simulink model "aero_dap3dof"  (R2021b)
settings: Solver=ode45  StartTime=0  StopTime=300  FixedStep=clockt/4  RelTol=1e-3  AbsTol=1e-6
PreLoadFcn:
  | run('aero_dap3dofdata.m');
undefined symbols (not defined in the file): alph1, alphs1, DB, deg, delt, euler_0, Force, L_arm, mass_0, pqr_0, r_moon_eq, rad, s
libraries: aerolibconvert2 x6, vrlib x2, aerolib6dof2 x1, sharedtransform x1, aerolibutil x1, aerolibgravity2 x1, aero_libdap x1, aero_librcs x1, commchan3 x1
CloseFcn:
  | h=findobj('type','figure','Name','aero_dap3dof');if ~isempty(h);close(h);end
Description:
  | Apollo Lunar Module Digital Autopilot
  | 
  | This model was featured in "Fly Me to the Moon - Then and Now", the story of the digital
  | autopilot in the Lunar Module from the Summer 1999 issue of "MATLAB(R) News & Notes".
  | Double click on the link in the model to view the article online over the Internet.
settings Model: RequirementInfo=9  Creator=The MathWorks, Inc.  LastModifiedBy=dev
settings SolverCC: AutoScaleAbsTol=off  AlgebraicLoopSolver=TrustRegion
settings DataIOCC: SaveFormat=Array  ReturnWorkspaceOutputs=off  SignalLoggingName=logsOut
settings OptimizationCC: BlockReduction=off  ExpressionDepthLimit=2147483647  InitFltsAndDblsToZero=on
settings DebuggingCC: SaveWithParameterizedLinksMsg=none  SignalResolutionControl=TryResolveAllWithWarning  MultiTaskDSMMsg=warning  MultiTaskCondExecSysMsg=none  SigSpecEnsureSampleTimeMsg=none  FcnCallInpInsideContextMsg=warning  StateNameClashWarn=warning  SFUnexpectedBacktrackingDiag=warning  SFNoUnconditionalDefaultTransitionDiag=warning  SFExecutionAtInitializationDiag=none  SFMachineParentedDataDiag=warning  ArithmeticOperatorsInVariantConditions=warning
settings HardwareCC: ProdBitPerPointer=32  ProdBitPerSizeT=32  ProdBitPerPtrDiffT=32  ProdLargestAtomicFloat=None  ProdIntDivRoundTo=Undefined  ProdEndianess=Unspecified  ProdWordSize=32  ProdHWDeviceType=Specified
settings ModelReferenceCC: PropagateSignalLabelsOutOfModel=off
settings SFSimCC: SimUseLocalCustomCode=off  SimParseCustomCode=off  CustomCodeUndefinedFunction=UseInterfaceOnly
settings RTWCC: RTWUseLocalCustomCode=off
settings CodeAppCC: StateflowObjectComments=on
settings GRTTargetCC: TargetLangStandard=C89/C90 (ANSI)
settings ConfigComp: CovMetricSettings=d  CovSaveCumulativeToWorkspaceVar=on  CovSaveSingleToWorkspaceVar=on  CovExternalEMLEnable=off

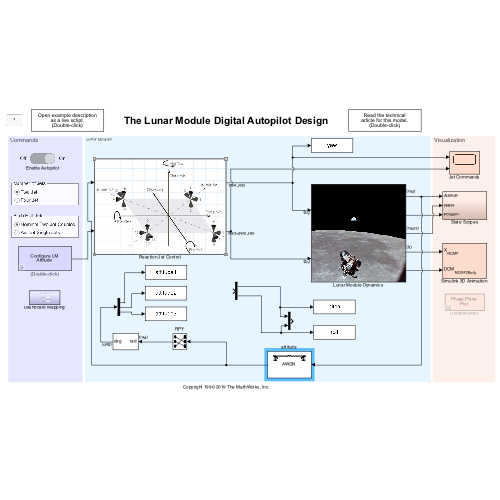
[thumbnail: Simulink's stored preview of the top-level diagram]
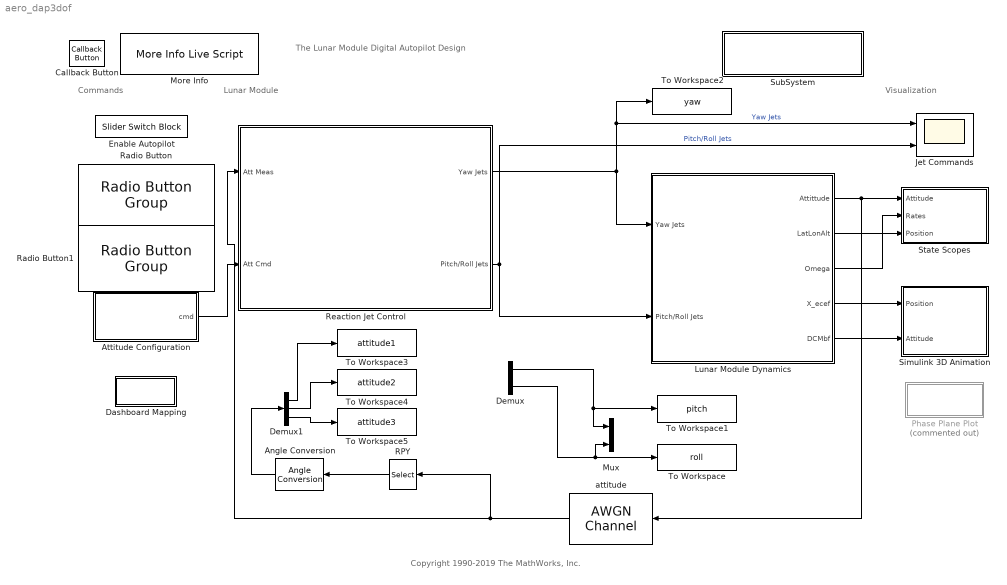
== system aero_dap3dof ==
  note: Lunar Module
  note: Visualization
  note: Commands
  note: The Lunar Module Digital Autopilot Design
  note: Copyright 1990-2019 The MathWorks, Inc.
  Angle Conversion : aerolibconvert2/Angle Conversion  IU=rad  OU=deg
  Attitude Configuration : Subsystem  mask(Configure LM Attitude){att_cmd=euler_0 + [2.87 5.73 0.606], p_0=0.573, q_0=0.573, r_0=6.808}
      mask prompts: att_cmd "<html>Pilot commanded<br>attitude (roll, pitch, yaw)<br>[deg, deg, deg]</html>"; p_0 "Roll rate [deg/s]"; q_0 "Pitch rate [deg/s]"; r_0 "Yaw rate [deg/s]"
      settings: AttributesFormatString=(Double-click)
      mask Callback p_0:
      | assignin('base', 'pqr_0', [str2double(get_param(gcb, 'p_0')),...
      |     str2double(get_param(gcb, 'q_0')), str2double(get_param(gcb, 'r_0'))]);
      mask Callback q_0:
      | assignin('base', 'pqr_0', [str2double(get_param(gcb, 'p_0')),...
      |     str2double(get_param(gcb, 'q_0')), str2double(get_param(gcb, 'r_0'))]);
      mask Callback r_0:
      | assignin('base', 'pqr_0', [str2double(get_param(gcb, 'p_0')),...
      |     str2double(get_param(gcb, 'q_0')), str2double(get_param(gcb, 'r_0'))]);
      mask DialogControl DescGroupVar1 Prompt: Pilot Commanded Body Attitude
      mask DialogControl DescTextVar_copy Prompt: Specify desired body attitude angles to send to digital autopilot.
      mask DialogControl ParameterGroupVar Prompt: Initial Body Angular Rates
      mask DialogControl DescTextVar Prompt: Vary the initial angular rates of the Lunar Module to investigate the response of the digital autopilot design.
      mask Display: disp('Configure LM\nAttitude')
  Callback Button : CallbackButton  ButtonText=?
      settings: ClickFcn=showExample('simulink_aerospace/DevelopingTheApolloLunarModuleDigitalAutopilotExample')
  Dashboard Mapping : Subsystem
  Demux : Demux  Outputs=2
  Demux1 : Demux  Outputs=3
  Enable Autopilot : SliderSwitchBlock  LabelPosition=Hide
      settings: Values={{'Off', 'On'}, [0 1]}
  Jet Commands : Scope  NumInputPorts=2
  Lunar Module Dynamics : Subsystem
      mask Display: image('$imagefile'); % Use "Edit Image" on toolstrip to change.
  More Info : aero_libdap/More Info Live Script  SystemSampleTime=-1  VariantActivationTime=update diagram  Latency=0  AutoFrameSizeCalculation=off
      settings: SourceProductBaseCode=SL
  Mux : Mux  Inputs=2
  Phase Plane Plot : Subsystem  Commented=on  mask(Phase Plane Plot){enablePlot=off}
      mask prompts: enablePlot "Enable yaw phase plane plot"
      mask help: Enable yaw phase plane plotting during simulation.
      settings: AttributesFormatString=(Double-click)
      settings: OpenFcn=|
      | if ~builtin('license','test','virtual_reality_toolbox')
      |     set_param(gcb, 'enableVis', 'off');
      | end
      | open_system(gcb,'mask');
      mask Callback enablePlot:
      | if strcmp(get_param(gcb,'enablePlot'), 'on')
      |     set_param(gcb, 'Commented', 'off');
      | else
      |     set_param(gcb, 'Commented', 'on');
      | end
      mask Display: disp('Phase Plane\nPlot')
  RPY : Selector  InputPortWidth=3  IndexOptions=Index vector (dialog)  Indices=[2 3 1]  OutputSizes=1
  Radio Button : RadioButtonGroup  LabelPosition=Hide  SelectedLabel=Two Jet  ButtonGroupName=Number of Jets
      settings: Values={{'Two Jet', 'Four Jet'}, [2 4]}
  Radio Button1 : RadioButtonGroup  LabelPosition=Hide  SelectedLabel=Nominal Two Jet Couples  ButtonGroupName=Pitch Roll Jets
      settings: Values={{'Nominal Two Jet Couples', 'Ascent Single Jets'}, [2 1]}
  Reaction Jet Control : Subsystem
      mask Display: image('$imagefile'); % Use "Edit Image" on toolstrip to change.
  Simulink 3D Animation : Subsystem  mask(Set Animation Properties){enableVis=on, visSampleTime=1}
      mask prompts: enableVis "Enable visualization with Simulink 3D Animation"; visSampleTime "Animation refresh rate:"
      mask help:
      | Change visualization properties used by Simulink 3D Animation. These settings are graphical only and do not affect simulation behavior.
      |
      | Hover over a dialog box for an explanation of the property.
      settings: OpenFcn=|
      | if ~builtin('license','test','virtual_reality_toolbox')
      |     set_param(gcb, 'enableVis', 'off');
      | end
      | open_system(gcb,'mask');
      mask Callback enableVis:
      | if strcmp(get_param(gcb,'enableVis'), 'on')
      |     enable = {'on', 'on'};
      |     set_param(gcb, 'Commented', 'off');
      | else
      |     enable = {'on', 'off'};
      |     set_param(gcb, 'Commented', 'on');
      | end
      | set_param(gcb,'MaskEnables', enable);
      | clear enable
      mask DialogControl vrOpenBtn Prompt: Open Simulink 3D Animation window
      mask DialogControl vrOpenBtn Callback: vrmfunc('FnOpen',getSimulinkBlockHandle([gcb '/VR Sink']));
      mask DialogControl visSampleTime Tooltip: <html>Sample time of animation window. Use this property to effectively speed up or slow down the animation. For example, a sample time of 1 causes the animation to update at every simulation time step. For a sample time of 20, the visualization will update every twentieth simulation time step. Maximum value is 1000.</html>
      mask Display:
      | port_label('input', 1, 'X_{MCMF}','texmode','on')
      | port_label('input', 2, 'DCM_{MCMF2Body}','texmode','on')
  State Scopes : Subsystem
  SubSystem : Subsystem
      mask init:
      | dispstr = sprintf('Read the technical\narticle for this model.\n(Double-click)');
      settings: OpenFcn=web('https://www.mathworks.com/company/newsletters/articles/the-apollo-11-moon-landing-spacecraft-design-then-and-now.html')
      mask Display: disp(dispstr)
  To Workspace : ToWorkspace  VariableName=roll  SampleTime=-1
      settings: Save2DSignal=2-D array (concatenate along first dimension)
  To Workspace1 : ToWorkspace  VariableName=pitch  SampleTime=-1
      settings: Save2DSignal=2-D array (concatenate along first dimension)
  To Workspace2 : ToWorkspace  VariableName=yaw  SampleTime=-1
      settings: Save2DSignal=2-D array (concatenate along first dimension)
  To Workspace3 : ToWorkspace  VariableName=attitude1  SampleTime=-1
      settings: Save2DSignal=2-D array (concatenate along first dimension)
  To Workspace4 : ToWorkspace  VariableName=attitude2  SampleTime=-1
  To Workspace5 : ToWorkspace  VariableName=attitude3  SampleTime=-1
      settings: Save2DSignal=2-D array (concatenate along first dimension)
  attitude : commchan3/AWGN Channel  InputProcessing=Columns as channels (frame based)  seed=67  noiseMode=Variance from mask  EbNodB=10  EsNodB=10  SNRdB=10  bitsPerSym=1  Ps=1  Tsym=1  variance=0.0000001
  wires:
  Attitude Configuration/1(cmd) -> Reaction Jet Control/2(Att Cmd)
  Lunar Module Dynamics/3(Omega) -> State Scopes/2(Rates)
  Lunar Module Dynamics/4(X_ecef) -> Simulink 3D Animation/1(Position)
  Lunar Module Dynamics/5(DCMbf) -> Simulink 3D Animation/2(Attitude)
  Reaction Jet Control/2(Pitch/Roll Jets) -> Lunar Module Dynamics/2(Pitch/Roll Jets), Jet Commands/2  "Pitch/Roll Jets"
  Demux/1 -> Mux/1, To Workspace1/1
  Lunar Module Dynamics/2(LatLonAlt) -> State Scopes/3(Position)
  Demux/2 -> Mux/2, To Workspace/1
  Lunar Module Dynamics/1(Attittude) -> State Scopes/1(Attitude), attitude/1
  RPY/1 -> Angle Conversion/1
  Angle Conversion/1 -> Demux1/1
  Reaction Jet Control/1(Yaw Jets) -> Lunar Module Dynamics/1(Yaw Jets), Jet Commands/1, To Workspace2/1  "Yaw Jets"
  attitude/1 -> Reaction Jet Control/1(Att Meas), RPY/1
  Demux1/1 -> To Workspace3/1
  Demux1/2 -> To Workspace4/1
  Demux1/3 -> To Workspace5/1

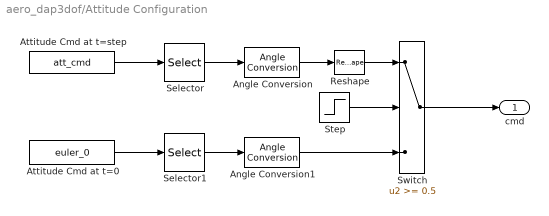
== system aero_dap3dof/Attitude Configuration ==
  Angle Conversion : aerolibconvert2/Angle Conversion  IU=deg  OU=rad
  Angle Conversion1 : aerolibconvert2/Angle Conversion  IU=deg  OU=rad
  Attitude Cmd at t=0 : Constant  Value=euler_0  VectorParams1D=off
  Attitude Cmd at t=step : Constant  Value=att_cmd  VectorParams1D=off
  Reshape : Reshape
  Selector : Selector  InputPortWidth=3  IndexOptions=Index vector (dialog)  Indices=[3 1 2]  OutputSizes=1
  Selector1 : Selector  InputPortWidth=3  IndexOptions=Index vector (dialog)  Indices=[3 1 2]  OutputSizes=1
  Step : Step  Time=.25  SampleTime=0
  Switch : Switch  Threshold=0.5  SaturateOnIntegerOverflow=on  InputSameDT=on
  cmd : Outport  VectorParamsAs1DForOutWhenUnconnected=off
  wires:
  Reshape/1 -> Switch/1
  Angle Conversion/1 -> Reshape/1
  Step/1 -> Switch/2
  Attitude Cmd at t=0/1 -> Selector1/1
  Selector/1 -> Angle Conversion/1
  Switch/1 -> cmd/1
  Selector1/1 -> Angle Conversion1/1
  Angle Conversion1/1 -> Switch/3
  Attitude Cmd at t=step/1 -> Selector/1

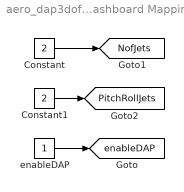
== system aero_dap3dof/Dashboard Mapping ==
  Constant : Constant  Value=2
  Constant1 : Constant  Value=2
  enableDAP : Constant
  tag scope: NofJets=global, PitchRollJets=global, enableDAP=global
  wires:
  Constant/1 -> [NofJets]
  Constant1/1 -> [PitchRollJets]
  enableDAP/1 -> [enableDAP]

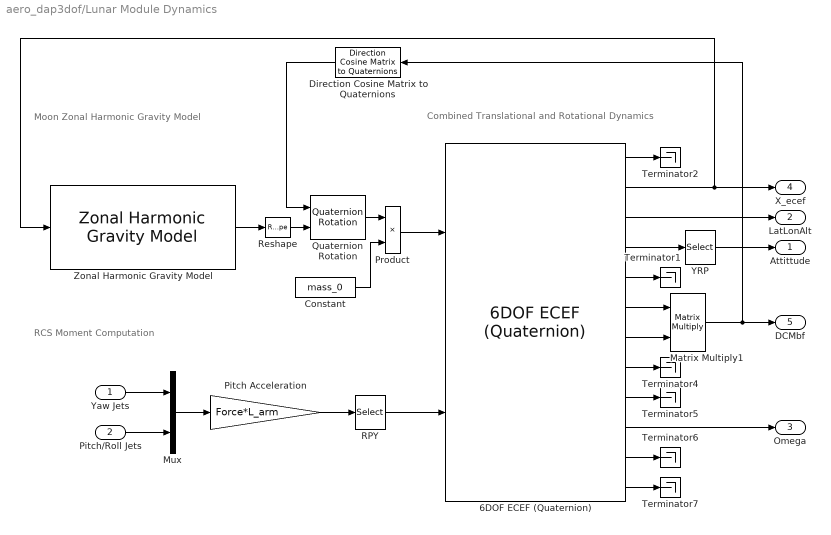
== system aero_dap3dof/Lunar Module Dynamics ==
  note: RCS Moment Computation
  note: Combined Translational and Rotational Dynamics
  note: Moon Zonal Harmonic Gravity Model
  Yaw Jets : Inport  Unit=lbf
  Pitch/Roll Jets : Inport  Port=2  Unit=lbf
  6DOF ECEF (Quaternion) : aerolib6dof2/6DOF ECEF (Quaternion)  units=English (Velocity in ft/s)  mtype=Fixed  xg_0=lla_0  Vm_0=vel_0  eul_0=euler_0*pi/180  pm_0=pqr_0*pi/180  mass_0=mass_0  mass_e=0.5  mass_f=2.0  inertia=Inertia_0  inertia_e=eye(3)  inertia_f=2*eye(3)  vre_flag=on  abi_flag=off  ptype=Custom  R=r_moon_eq  F=f_moon  w_E=omega_moon  angle_in=Internal  LG0=0  quat_statename=''  pm_statename=''  Vm_statename=''  posECEF_statename=''  posECI_statename=''  LG_statename=''  mass_statename=''
      settings: SourceProductBaseCode=AE
  Constant : Constant  Value=mass_0
  Direction Cosine Matrix to Quaternions : sharedtransform/Direction Cosine Matrix  to Quaternions  aMode=0  action=None  tolerance=eps(2)
      settings: SourceProductBaseCode=AE,PW,DR,MT,UV,VE
  Matrix Multiply1 : Product  Multiplication=Matrix(*)
  Mux : Mux  Inputs=2
  Pitch Acceleration : Gain  Gain=Force*L_arm  SaturateOnIntegerOverflow=on  OutDataTypeStr=Inherit: Same as input  ParamDataTypeStr=Inherit: Same as input
  Product : Product
  Quaternion Rotation : aerolibutil/Quaternion Rotation
  RPY : Selector  InputPortWidth=3  IndexOptions=Index vector (dialog)  Indices=[2 3 1]  OutputSizes=1
  Reshape : Reshape
  Terminator{1..2,4..7} (6 alike) : Terminator
  YRP : Selector  InputPortWidth=3  IndexOptions=Index vector (dialog)  Indices=[3 1 2]  OutputSizes=1
  Zonal Harmonic Gravity Model : aerolibgravity2/Zonal Harmonic Gravity Model  units=English  degree=2  action=Warning  ptype=Moon  R=5702099.7375  GM=173140712687447.5  jvalue=[2.0270000e-04]
      settings: SourceProductBaseCode=AE
  Attittude : Outport  Unit=rad  VectorParamsAs1DForOutWhenUnconnected=off
  LatLonAlt : Outport  Port=2  VectorParamsAs1DForOutWhenUnconnected=off
  Omega : Outport  Port=3  Unit=rad/s  VectorParamsAs1DForOutWhenUnconnected=off
  X_ecef : Outport  Port=4  Unit=ft  VectorParamsAs1DForOutWhenUnconnected=off
  DCMbf : Outport  Port=5  VectorParamsAs1DForOutWhenUnconnected=off
  wires:
  Pitch/Roll Jets/1 -> Mux/2
  Yaw Jets/1 -> Mux/1
  Mux/1 -> Pitch Acceleration/1
  6DOF ECEF (Quaternion)/4 -> YRP/1
  6DOF ECEF (Quaternion)/10 -> Omega/1
  Matrix Multiply1/1 -> Direction Cosine Matrix to Quaternions/1, DCMbf/1
  6DOF ECEF (Quaternion)/6 -> Matrix Multiply1/1
  6DOF ECEF (Quaternion)/7 -> Matrix Multiply1/2
  Zonal Harmonic Gravity Model/1 -> Reshape/1
  Quaternion Rotation/1 -> Product/1
  Reshape/1 -> Quaternion Rotation/2
  Direction Cosine Matrix to Quaternions/1 -> Quaternion Rotation/1
  6DOF ECEF (Quaternion)/1 -> Terminator2/1
  6DOF ECEF (Quaternion)/5 -> Terminator1/1
  6DOF ECEF (Quaternion)/2 -> X_ecef/1, Zonal Harmonic Gravity Model/1
  6DOF ECEF (Quaternion)/9 -> Terminator5/1
  6DOF ECEF (Quaternion)/8 -> Terminator4/1
  6DOF ECEF (Quaternion)/11 -> Terminator6/1
  6DOF ECEF (Quaternion)/12 -> Terminator7/1
  6DOF ECEF (Quaternion)/3 -> LatLonAlt/1
  Constant/1 -> Product/2
  Product/1 -> 6DOF ECEF (Quaternion)/1
  Pitch Acceleration/1 -> RPY/1
  RPY/1 -> 6DOF ECEF (Quaternion)/2
  YRP/1 -> Attittude/1

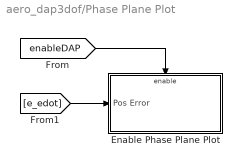
== system aero_dap3dof/Phase Plane Plot ==
  Enable Phase Plane Plot : Subsystem
  wires:
  [enableDAP] -> Enable Phase Plane Plot/Enable
  [e_edot] -> Enable Phase Plane Plot/1(Pos Error)

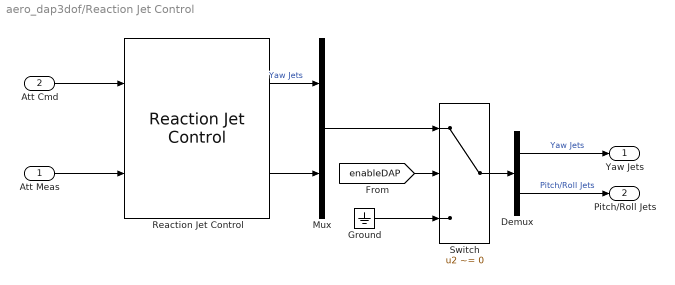
== system aero_dap3dof/Reaction Jet Control ==
  Att Meas : Inport
  Att Cmd : Inport  Port=2
  Demux : Demux  Outputs=[1 2]
  Ground : Ground
  Mux : Mux  Inputs=2
  Reaction Jet Control : aero_librcs/Reaction Jet Control  SystemSampleTime=-1  VariantActivationTime=update diagram  Latency=0  AutoFrameSizeCalculation=off
      settings: SourceProductBaseCode=SL
  Switch : Switch  Criteria=u2 ~= 0
  Yaw Jets : Outport  VectorParamsAs1DForOutWhenUnconnected=off
  Pitch/Roll Jets : Outport  Port=2  VectorParamsAs1DForOutWhenUnconnected=off
  wires:
  Att Cmd/1 -> Reaction Jet Control/1
  Att Meas/1 -> Reaction Jet Control/2
  Demux/1 -> Yaw Jets/1  "Yaw Jets"
  Demux/2 -> Pitch/Roll Jets/1  "Pitch/Roll Jets"
  Ground/1 -> Switch/3
  Reaction Jet Control/1 -> Mux/1  "Yaw Jets"
  [enableDAP] -> Switch/2
  Mux/1 -> Switch/1
  Reaction Jet Control/2 -> Mux/2
  Switch/1 -> Demux/1

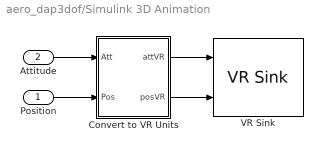
== system aero_dap3dof/Simulink 3D Animation ==
  Position : Inport
  Attitude : Inport  Port=2
  Convert to VR Units : Subsystem
  VR Sink : vrlib/VR Sink  InstantiateOnLoad=on  SampleTime=visSampleTime  ViewEnable=on  RemoteChange=off  RemoteView=off  FieldsWritten=LSAM.rotation.4.1.1.double#LSAM.translation.3.1.1.double  WorldFileName=Lander_Moon180_1.wrl  WorldDescription=Apollo Lunar Module Descent Animation  AutoView=on  VideoDimensions=[]  AllowVariableSize=off  FigureProperties="{'Position', 'Name', 'Viewpoint', 'CameraBound', 'CameraDirection', 'CameraPosition', 'CameraUpVector', 'ZoomFactor', 'Antialiasing', 'Headlight', 'Lighting', 'NavPanel', 'Sound', 'StatusBar', 'Stereo3D', 'Stereo3DCameraOffset', 'Stereo3DHIT', 'ToolBar', 'Textures', 'Transparency', 'Triad', 'Wireframe', 'NavZones', 'NavMode', 'NavSpeed', 'CaptureFileFormat', 'CaptureFileName', 'Record2DCompressMethod', 'Record2DCompressQuality', 'Record2D', 'Record2DFileName', 'Record2DFPS'; [5.0000000000000000e+00   1.0300000000000000e+02   5.7600000000000000e+02   3.5000000000000000e+02], 'Apollo Lunar Module Descent Animation', 'Follow Lander 1', 'on', [0.0000000000000000e+00   0.0000000000000000e+00  -1.0000000000000000e+00], [0.0000000000000000e+00   0.0000000000000000e+00   0.0000000000000000e+00], [0.0000000000000000e+00   1.0000000000000000e+00   0.0000000000000000e+00], [1.0000000000000000e+00], 'on', 'on', 'on', 'halfbar', 'on', 'on', 'off', [1.0000000149011612e-01], [0.0000000000000000e+00], 'on', 'on', 'on', 'none', 'off', 'off', 'fly', 'normal', 'tif', '%f_anim_%n.tif', 'auto', [7.5000000000000000e+01], 'off', '%f_anim_%n.avi', 'auto'}"
  wires:
  Attitude/1 -> Convert to VR Units/1(Att)
  Position/1 -> Convert to VR Units/2(Pos)
  Convert to VR Units/1(attVR) -> VR Sink/1
  Convert to VR Units/2(posVR) -> VR Sink/2

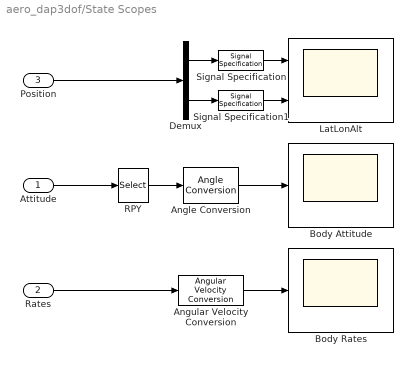
== system aero_dap3dof/State Scopes ==
  Attitude : Inport
  Rates : Inport  Port=2
  Position : Inport  Port=3
  Angle Conversion : aerolibconvert2/Angle Conversion  IU=rad  OU=deg
  Angular Velocity Conversion : aerolibconvert2/Angular Velocity Conversion  IU=rad/s  OU=deg/s
  Body Attitude : Scope
  Body Rates : Scope
  Demux : Demux  Outputs=[2 1]
  LatLonAlt : Scope  NumInputPorts=2
  RPY : Selector  InputPortWidth=3  IndexOptions=Index vector (dialog)  Indices=[2 3 1]  OutputSizes=1
  Signal Specification : SignalSpecification  Unit=deg
  Signal Specification1 : SignalSpecification  Unit=ft
  wires:
  Attitude/1 -> RPY/1
  Rates/1 -> Angular Velocity Conversion/1
  Demux/2 -> Signal Specification1/1
  Demux/1 -> Signal Specification/1
  Angle Conversion/1 -> Body Attitude/1
  Angular Velocity Conversion/1 -> Body Rates/1
  Signal Specification/1 -> LatLonAlt/1
  Signal Specification1/1 -> LatLonAlt/2
  RPY/1 -> Angle Conversion/1
  Position/1 -> Demux/1

== system aero_dap3dof/SubSystem ==

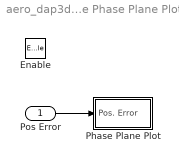
== system aero_dap3dof/Phase Plane Plot/Enable Phase Plane Plot ==
  Pos Error : Inport
  Enable : EnablePort  StatesWhenEnabling=reset
  Phase Plane Plot : Subsystem
  wires:
  Pos Error/1 -> Phase Plane Plot/1(Pos. Error)

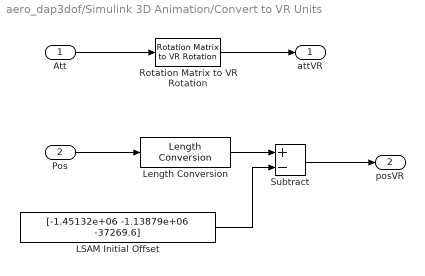
== system aero_dap3dof/Simulink 3D Animation/Convert to VR Units ==
  Att : Inport
  Pos : Inport  Port=2
  "LSAM Initial Offset " : Constant  Value=[-1.45132e+06 -1.13879e+06 -37269.6]
  Length Conversion : aerolibconvert2/Length Conversion  IU=ft  OU=m
  Rotation Matrix to VR Rotation : vrlib/Utilities/Rotation Matrix to VR Rotation  maxzero=1e-12
      settings: SourceProductBaseCode=SL
  Subtract : Sum  Inputs=+-
  attVR : Outport  VectorParamsAs1DForOutWhenUnconnected=off
  posVR : Outport  Port=2  VectorParamsAs1DForOutWhenUnconnected=off
  wires:
  Att/1 -> Rotation Matrix to VR Rotation/1
  Rotation Matrix to VR Rotation/1 -> attVR/1
  Pos/1 -> Length Conversion/1
  Length Conversion/1 -> Subtract/1
  Subtract/1 -> posVR/1
  "LSAM Initial Offset "/1 -> Subtract/2

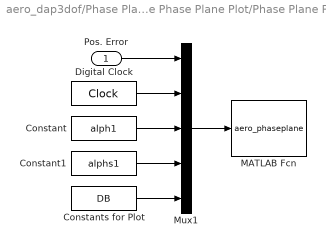
== system aero_dap3dof/Phase Plane Plot/Enable Phase Plane Plot/Phase Plane Plot ==
  Pos. Error : Inport
  Constant : Constant  Value=alph1
  Constant1 : Constant  Value=alphs1
  Constants for Plot : Constant  Value=DB
  Digital Clock : DigitalClock  SampleTime=delt
  MATLAB Fcn : MATLABFcn  MATLABFcn=aero_phaseplane  OutputDimensions=0
  Mux1 : Mux  Inputs=5
  wires:
  Mux1/1 -> MATLAB Fcn/1
  Pos. Error/1 -> Mux1/1
  Digital Clock/1 -> Mux1/2
  Constants for Plot/1 -> Mux1/5
  Constant/1 -> Mux1/3
  Constant1/1 -> Mux1/4
